simulink model "AMR_MoboticStartup_23b"  (R2024a)
settings: Solver=FixedStepDiscrete  StartTime=0.0  StopTime=inf  FixedStep=1e-3  RelTol=1e-3
model workspace (MAT data in the model file):
  mdlWSDbList = "C:\Users\matlab.cut\Desktop\AMR\canbus_files\tramontina_database_mobotic.dbc"
  mobotic_mechanical_offset = -30
settings Model: SimulationMode=external  Creator=matlab.cut  LastModifiedBy=matlab.cut
settings SolverCC: ConcurrentTasks=on  PositivePriorityOrder=on  AutoInsertRateTranBlk=on
settings OptimizationCC: BlockReduction=off  DefaultParameterBehavior=Inlined  OptimizeBlockIOStorage=off
settings DebuggingCC: TasksWithSamePriorityMsg=none
settings HardwareCC: ProdBitPerLong=64  ProdLongLongMode=on  ProdHWDeviceType=Intel->x86-64 (Linux 64)
settings ModelReferenceCC: ModelReferenceNumInstancesAllowed=Single
settings SFSimCC: MATLABDynamicMemAlloc=off
settings RTWCC: Description=Speedgoat Real-Time Target Machine  SystemTargetFile=speedgoat.tlc  TemplateMakefile=slrealtime_default_tmf  Toolchain=Simulink Real-Time Toolchain  BuildConfiguration=Faster Runs  CodeExecutionProfiling=on  TargetLang=C++  GPUComputeCapability=3.5
settings CodeAppCC: MaxIdLength=127
settings SimulinkRealTimeTargetCC: InstructionSetFMA=off  LogToMDFFile=off

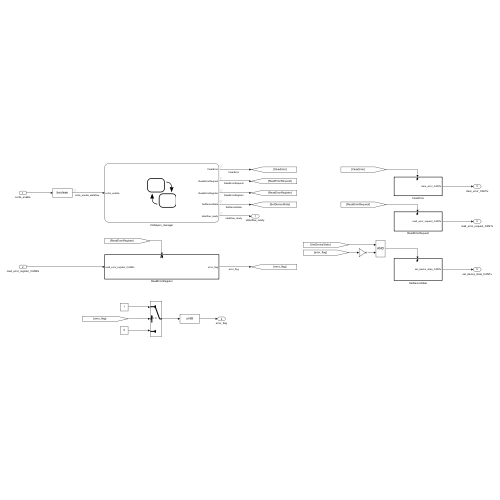
[thumbnail: Simulink's stored preview of the top-level diagram]
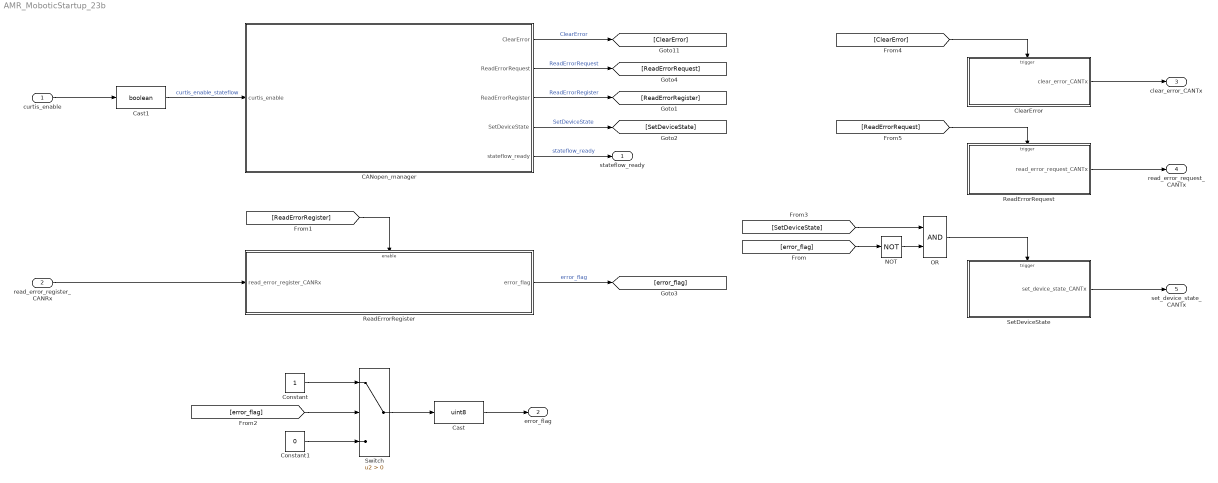
== system AMR_MoboticStartup_23b ==
  curtis_enable : Inport
  read_error_register_CANRx : Inport  Port=2
  CANopen_manager : Stateflow chart  TreatAsAtomicUnit=on
  Cast : DataTypeConversion  OutDataTypeStr=uint8  SaturateOnIntegerOverflow=off  RndMeth=Floor
  Cast1 : DataTypeConversion  OutDataTypeStr=boolean  SaturateOnIntegerOverflow=off  RndMeth=Floor
  ClearError : Subsystem  TreatAsAtomicUnit=on
  Constant : Constant
  Constant1 : Constant  Value=0
  NOT : Logic  Operator=NOT  IconShape=distinctive  AllPortsSameDT=off  OutDataTypeStr=boolean
  OR : Logic  AllPortsSameDT=off  OutDataTypeStr=boolean
  ReadErrorRegister : Subsystem  TreatAsAtomicUnit=on
  ReadErrorRequest : Subsystem  TreatAsAtomicUnit=on
  SetDeviceState : Subsystem  TreatAsAtomicUnit=on
  Switch : Switch  Criteria=u2 > Threshold  SaturateOnIntegerOverflow=off  InputSameDT=off
  stateflow_ready : Outport
  error_flag : Outport  Port=2
  clear_error_CANTx : Outport  Port=3
  read_error_request_CANTx : Outport  Port=4
  set_device_state_CANTx : Outport  Port=5
  wires:
  CANopen_manager/1(ClearError) -> [ClearError]  "ClearError"
  CANopen_manager/4(SetDeviceState) -> [SetDeviceState]  "SetDeviceState"
  CANopen_manager/3(ReadErrorRegister) -> [ReadErrorRegister]  "ReadErrorRegister"
  [error_flag] -> Switch/2
  Switch/1 -> Cast/1
  Cast/1 -> error_flag/1
  [SetDeviceState] -> OR/1
  [error_flag] -> NOT/1
  curtis_enable/1 -> Cast1/1
  Cast1/1 -> CANopen_manager/1(curtis_enable)  "curtis_enable_stateflow"
  Constant/1 -> Switch/1
  Constant1/1 -> Switch/3
  ReadErrorRegister/1(error_flag) -> [error_flag]  "error_flag"
  CANopen_manager/5(stateflow_ready) -> stateflow_ready/1  "stateflow_ready"
  NOT/1 -> OR/2
  CANopen_manager/2(ReadErrorRequest) -> [ReadErrorRequest]  "ReadErrorRequest"
  [ReadErrorRegister] -> ReadErrorRegister/Enable
  ClearError/1(clear_error_CANTx) -> clear_error_CANTx/1
  read_error_register_CANRx/1 -> ReadErrorRegister/1(read_error_register_CANRx)
  SetDeviceState/1(set_device_state_CANTx) -> set_device_state_CANTx/1
  ReadErrorRequest/1(read_error_request_CANTx) -> read_error_request_CANTx/1
  [ClearError] -> ClearError/Trigger
  [ReadErrorRequest] -> ReadErrorRequest/Trigger
  OR/1 -> SetDeviceState/Trigger

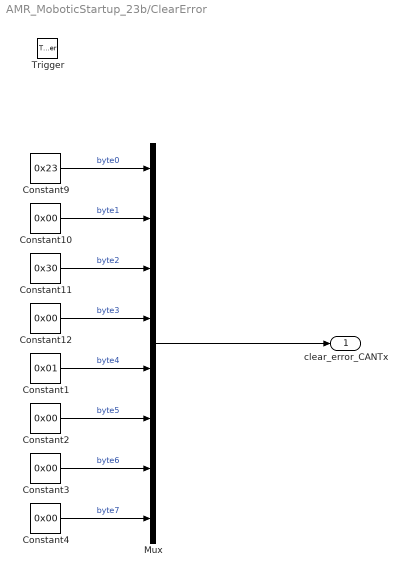
== system AMR_MoboticStartup_23b/ClearError ==
  Trigger : TriggerPort  VariantControl=(inherit)  PortDimensions=1
  Constant1 : Constant  Value=0x01
  Constant{2..4,10,12} (5 alike) : Constant  Value=0x00
  Constant11 : Constant  Value=0x30
  Constant9 : Constant  Value=0x23
  Mux : Mux  Inputs=8
  clear_error_CANTx : Outport  OutputWhenDisabled=reset  InitialOutput=0
  wires:
  Mux/1 -> clear_error_CANTx/1
  Constant4/1 -> Mux/8  "byte7"
  Constant9/1 -> Mux/1  "byte0"
  Constant10/1 -> Mux/2  "byte1"
  Constant11/1 -> Mux/3  "byte2"
  Constant12/1 -> Mux/4  "byte3"
  Constant1/1 -> Mux/5  "byte4"
  Constant2/1 -> Mux/6  "byte5"
  Constant3/1 -> Mux/7  "byte6"

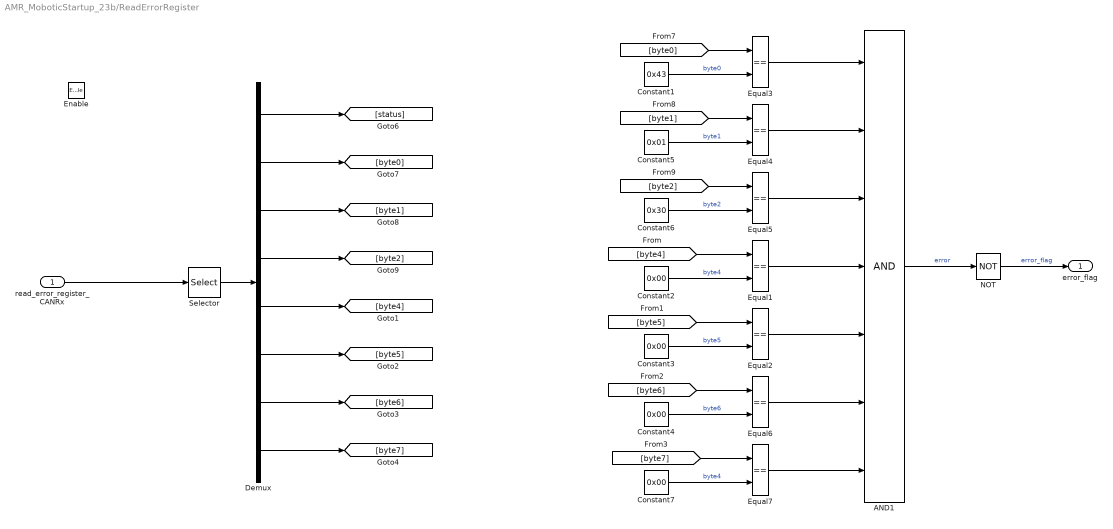
== system AMR_MoboticStartup_23b/ReadErrorRegister ==
  read_error_register_CANRx : Inport
  Enable : EnablePort  StatesWhenEnabling=reset
  AND1 : Logic  Inputs=7  AllPortsSameDT=off  OutDataTypeStr=boolean
  Constant1 : Constant  Value=0x43
  Constant{2..4,7} (4 alike) : Constant  Value=0x00
  Constant5 : Constant  Value=0x01
  Constant6 : Constant  Value=0x30
  Demux : Demux  Outputs=8
  Equal{1..7} (7 alike) : RelationalOperator  Operator===  OutDataTypeStr=boolean  RndMeth=Simplest  InputSameDT=off
  NOT : Logic  Operator=NOT  IconShape=distinctive  AllPortsSameDT=off  OutDataTypeStr=boolean
  Selector : Selector  IndexMode=Zero-based  InputPortWidth=9  IndexOptions=Index vector (dialog)  Indices=[0:3,5:8]  OutputSizes=1
  error_flag : Outport  InitialOutput=[0]
  wires:
  [byte0] -> Equal3/1
  Constant5/1 -> Equal4/2  "byte1"
  [byte1] -> Equal4/1
  [byte2] -> Equal5/1
  Demux/8 -> [byte7]
  Demux/4 -> [byte2]
  Demux/2 -> [byte0]
  Demux/1 -> [status]
  Demux/7 -> [byte6]
  Demux/6 -> [byte5]
  read_error_register_CANRx/1 -> Selector/1
  Demux/5 -> [byte4]
  Constant6/1 -> Equal5/2  "byte2"
  Demux/3 -> [byte1]
  Constant1/1 -> Equal3/2  "byte0"
  Constant2/1 -> Equal1/2  "byte4"
  [byte4] -> Equal1/1
  [byte5] -> Equal2/1
  Constant3/1 -> Equal2/2  "byte5"
  Constant4/1 -> Equal6/2  "byte6"
  [byte6] -> Equal6/1
  [byte7] -> Equal7/1
  Constant7/1 -> Equal7/2  "byte4"
  AND1/1 -> NOT/1  "error"
  NOT/1 -> error_flag/1  "error_flag"
  Equal3/1 -> AND1/1
  Equal4/1 -> AND1/2
  Equal5/1 -> AND1/3
  Equal1/1 -> AND1/4
  Equal2/1 -> AND1/5
  Equal6/1 -> AND1/6
  Equal7/1 -> AND1/7
  Selector/1 -> Demux/1

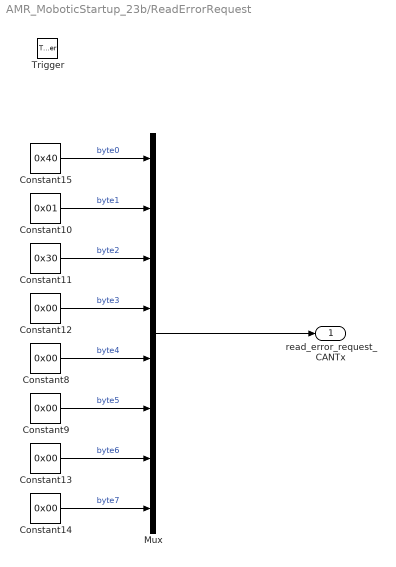
== system AMR_MoboticStartup_23b/ReadErrorRequest ==
  Trigger : TriggerPort  VariantControl=(inherit)  PortDimensions=1
  Constant10 : Constant  Value=0x01
  Constant11 : Constant  Value=0x30
  Constant{8..9,12..14} (5 alike) : Constant  Value=0x00
  Constant15 : Constant  Value=0x40
  Mux : Mux  Inputs=8
  read_error_request_CANTx : Outport  OutputWhenDisabled=reset  InitialOutput=0
  wires:
  Constant11/1 -> Mux/3  "byte2"
  Constant9/1 -> Mux/6  "byte5"
  Constant14/1 -> Mux/8  "byte7"
  Constant15/1 -> Mux/1  "byte0"
  Mux/1 -> read_error_request_CANTx/1
  Constant10/1 -> Mux/2  "byte1"
  Constant12/1 -> Mux/4  "byte3"
  Constant8/1 -> Mux/5  "byte4"
  Constant13/1 -> Mux/7  "byte6"

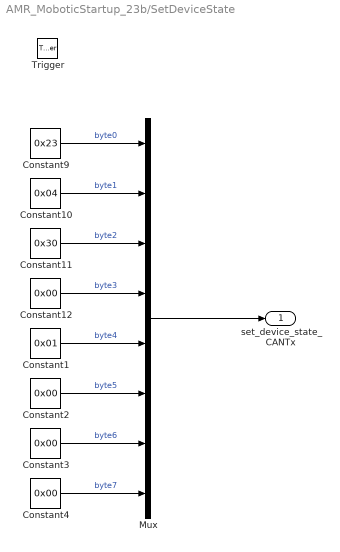
== system AMR_MoboticStartup_23b/SetDeviceState ==
  Trigger : TriggerPort  VariantControl=(inherit)  PortDimensions=1
  Constant1 : Constant  Value=0x01
  Constant10 : Constant  Value=0x04
  Constant11 : Constant  Value=0x30
  Constant{2..4,12} (4 alike) : Constant  Value=0x00
  Constant9 : Constant  Value=0x23
  Mux : Mux  Inputs=8
  set_device_state_CANTx : Outport  OutputWhenDisabled=reset  InitialOutput=0
  wires:
  Constant10/1 -> Mux/2  "byte1"
  Constant4/1 -> Mux/8  "byte7"
  Constant12/1 -> Mux/4  "byte3"
  Constant9/1 -> Mux/1  "byte0"
  Constant1/1 -> Mux/5  "byte4"
  Constant2/1 -> Mux/6  "byte5"
  Constant3/1 -> Mux/7  "byte6"
  Constant11/1 -> Mux/3  "byte2"
  Mux/1 -> set_device_state_CANTx/1

== stateflow chart AMR_MoboticStartup_23b/CANopen_manager ==
  settings: updateMethod=DISCRETE  sampleTime=5e-3
  state SetDeviceStateON
    entry:
    ClearError = 0; % send clear error command
    ReadErrorRegister = 0;
    ReadErrorRegister = 0;
    SetDeviceState = 1;
    stateflow_ready = 0;
    exit:
    SetDeviceState = 0;
  state idle
    entry:
    ClearError = 0; % send clear error command
    ReadErrorRequest = 0; % request to read error
    ReadErrorRegister = 0; % read error register
    SetDeviceState = 0; % send enable command
  state ReadErrorRegister
    entry:
    ClearError = 0;
    ReadErrorRequest = 0;
    ReadErrorRegister = 1;
    SetDeviceState = 0;
    stateflow_ready = 0;
  state wait_for_curtis
    entry:
    ClearError = 0; % send clear error command
    ReadErrorRequest = 0; % request to read error
    ReadErrorRegister = 0; % read error register
    SetDeviceState = 0; % send enable command
    exit:
    i = i+1;
  state ClearError
    entry:
    ClearError = 1;
    ReadErrorRequest = 0;
    ReadErrorRegister = 0;
    SetDeviceState = 0;
    stateflow_ready = 0;
    exit:
    ClearError = 0;
  state ReadErrorRequest
    entry:
    ClearError = 0;
    ReadErrorRequest = 1;
    ReadErrorRegister = 0;
    SetDeviceState = 0;
    stateflow_ready = 0;
    exit:
    ReadErrorRequest = 0;
  (default) -> idle : {i = 5; stateflow_ready = 0}
  idle -> idle [order 2]
  SetDeviceStateON -> idle : [after(20,msec)]
      | {stateflow_ready = 1}
  idle -> wait_for_curtis [order 1] : [curtis_enable == true] {i = 0; stateflow_ready = 0;}
  ReadErrorRegister -> SetDeviceStateON [order 1] : [i  == 3]
      | {ReadErrorRegister = 0}
  ReadErrorRegister -> wait_for_curtis [order 2] : [i < 3]
  wait_for_curtis -> ClearError : after(1,sec)
  ReadErrorRequest -> ReadErrorRegister : after(10,msec)
  ClearError -> ReadErrorRequest : after(10,msec)
  data: curtis_enable input; ClearError output; ReadErrorRequest output; ReadErrorRegister output; SetDeviceState output; stateflow_ready output; i local
